simulink model "BatteryHVDetailed_harness_model"  (R2022a)
settings: Solver=daessc  StartTime=0.0  StopTime=500  RelTol=1e-3  AbsTol=1e-3
PreLoadFcn:
  | BatteryHVDetailed_harness_params
  | 
  | load("BatteryHV_CurrentProfile.mat")
undefined symbols (not defined in the file or in its folder): Module, Multi
libraries: fl_lib x2, nesl_utility x2
settings Model: PacingRate=6  Creator=isaacito  LastModifiedBy=isaacito
settings SolverCC: AutoScaleAbsTol=off  AlgebraicLoopSolver=TrustRegion
settings DataIOCC: DSMLogging=off
settings DebuggingCC: UnconnectedInputMsg=warning  UnconnectedOutputMsg=warning  UnconnectedLineMsg=warning  SFMachineParentedDataDiag=warning
settings RTWCC: DLArmComputeVersion=19.05
settings SimscapeCC: SimscapeLogType=local  SimscapeLogSimulationStatistics=on  SimscapeLogToSDI=on  SimscapeLogLimitData=off

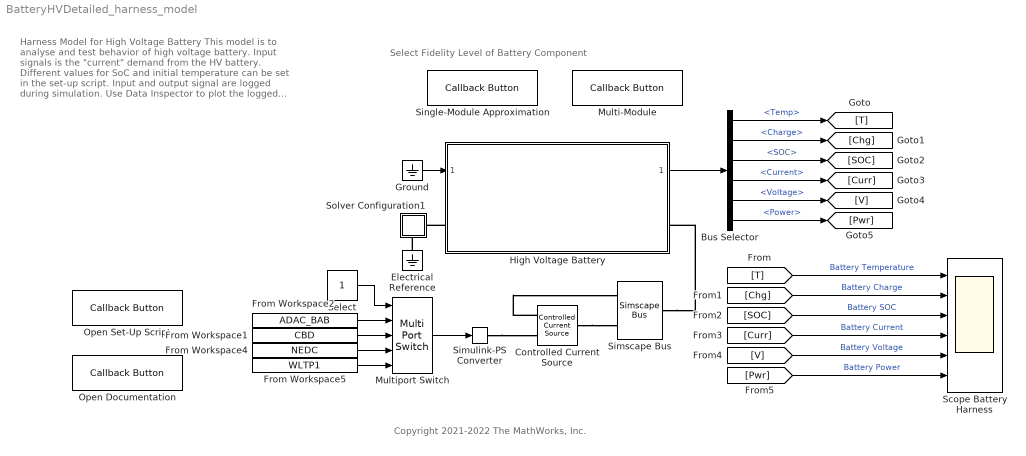
== system BatteryHVDetailed_harness_model ==
  note: Select Fidelity Level of Battery Component
  note: Copyright 2021-2022 The MathWorks, Inc.
  note: Harness Model for
      | High Voltage Battery
      |
      | This model is to analyse and test behavior of high voltage battery.
      |
      | Input signals is the "current" demand from the HV battery. Different values for SoC and initial temperature can be set in the set-up script.
      |
      | Input and output signal are logged during simulation. Use Data Inspector to plot the logged signals.
  " Simscape Bus" : SimscapeBus  HierarchyStrings=plus;minus
  Bus Selector : BusSelector  OutputSignals=Temp,Charge,SOC,Current,Voltage,Power
  Controlled Current Source : fl_lib/Electrical/Electrical Sources/Controlled Current Source
      settings: SourceProductBaseCode=PW,SS,VE
  Electrical Reference : fl_lib/Electrical/Electrical Elements/Electrical Reference
      settings: SourceProductBaseCode=PW,SS,VE
  From Workspace1 : FromWorkspace  VariableName=CBD
  From Workspace2 : FromWorkspace  VariableName=ADAC_BAB
  From Workspace4 : FromWorkspace  VariableName=NEDC
  From Workspace5 : FromWorkspace  VariableName=WLTP1
  Ground : Ground
  High Voltage Battery : Subsystem  ReferencedSubsystem=BatteryHVDetailed_refsub_SingleApprox
  Multi-Module : CallbackButton  ButtonText=Multi-Module
      settings: ClickFcn=|
      | disp("Selecting " + ...
      |   "multi-module component...")
      | 
      | set_param( gcs + "/High Voltage Battery", ...
      |   ReferencedSubsystem = ...
      |   "BatteryHVDetailed_refsub_MultiModule");
      | 
      | BatteryHVDetailed_params_MultiModule
      | 
      | load("BatteryHV_CurrentProfile.mat")
  Multiport Switch : MultiPortSwitch  Inputs=4  SaturateOnIntegerOverflow=off  InputSameDT=off
  Open Documentation : CallbackButton  ButtonText=Open Doc
      settings: ClickFcn=open('batteryModuleDoc_parameterDefinition.html')
  Open Set-Up Script : CallbackButton  ButtonText=Open Script
      settings: ClickFcn="edit(\"BatteryHVDetailed_harness_params\")"
  Scope Battery Harness : Scope  NumInputPorts=6
  Select : Constant
  Simulink-PS Converter : nesl_utility/Simulink-PS Converter  PhysicalDomain=network_engine_domain  SubClassName=ps_input  LeftPortType=input  RightPortType=output  PseudoPeriodic=off  Frequencies=[]  NoiseDistribution=none  NoiseParameters=[]  Unit=A  AffineConversion=off  FilteringAndDerivatives=provide  SimscapeFilterOrder=1  InputFilterTimeConstant=0.001  UdotUserProvided=0
      settings: SourceProductBaseCode=SS,PW,VE
  Single-Module Approximation : CallbackButton  ButtonText=Single-Module Approx.
      settings: ClickFcn=|
      | disp("Selecting " + ...
      |   "single-module approximation component...")
      | 
      | set_param( gcs + "/High Voltage Battery", ...
      |   ReferencedSubsystem = ...
      |   "BatteryHVDetailed_refsub_SingleApprox");
      | 
      | BatteryHVDetailed_params_SingleApprox
      | 
      | load("BatteryHV_CurrentProfile.mat")
  Solver Configuration1 : Subsystem
      settings: PortSchema="{\"entries\":[{\"content\":{\"sides\":[{\"content\":{\"connectorIds\":[]},\"type\":\"ConnectorPlacement.EquallySpacedRectSide\",\"uuid\":\"4a7e26c2-e9e9-4fea-b605-533b1a682be7\"},{\"content\":{\"connectorIds\":[\"RConn1\"],\"side\":\"RIGHT\"},\"type\":\"ConnectorPlacement.EquallySpacedRectSide\",\"uuid\":\"0210e324-555e-4372-b836-fcc8ab23e933\"},{\"content\":{\"connectorIds\":[],\"side\":\"TOP\"},\"type\":\"ConnectorPlacement.EquallySpacedRectSide\",\"uuid\":\"9bbae011-e6fc-4534-a44f-d79a5697c939\"},{\"content\":{\"connectorIds\":[\"RConn2\"],\"side\":\"BOTTOM\"},\"type\":\"ConnectorPlacement.EquallySpacedRectSide\",\"uuid\":\"d5829c0a-26ea-402d-a1c6-900997ddf1a8\"}]},\"type\":\"ConnectorPlacement.EquallySpacedConnector\",\"uuid\":\"f4e17c65-54c6-42fe-a467-9c6b014b697a\"}],\"packageUris\":[\"http://schema.mathworks.com/mf0/Connector/19700101\"],\"version\":\"1.0\"}"
  wires:
  Multiport Switch/1 -> Simulink-PS Converter/1
  From Workspace1/1 -> Multiport Switch/3
  From Workspace5/1 -> Multiport Switch/5
  From Workspace2/1 -> Multiport Switch/2
  Select/1 -> Multiport Switch/1
  From Workspace4/1 -> Multiport Switch/4
  Ground/1 -> High Voltage Battery/1
  High Voltage Battery/1 -> Bus Selector/1
  Bus Selector/1 -> [T]  "<Temp>"
  Bus Selector/2 -> [Chg]  "<Charge>"
  Bus Selector/3 -> [SOC]  "<SOC>"
  Bus Selector/4 -> [Curr]  "<Current>"
  Bus Selector/5 -> [V]  "<Voltage>"
  Bus Selector/6 -> [Pwr]  "<Power>"
  [T] -> Scope Battery Harness/1  "Battery Temperature"
  [Chg] -> Scope Battery Harness/2  "Battery Charge"
  [SOC] -> Scope Battery Harness/3  "Battery SOC"
  [Curr] -> Scope Battery Harness/4  "Battery Current"
  [V] -> Scope Battery Harness/5  "Battery Voltage"
  [Pwr] -> Scope Battery Harness/6  "Battery Power"
  connections:
  Electrical Reference/LConn1 -- Solver Configuration1/RConn2
  High Voltage Battery/LConn1 -- Solver Configuration1/RConn1
  " Simscape Bus"/RConn1 -- High Voltage Battery/RConn1
  Controlled Current Source/RConn2 -- " Simscape Bus"/LConn1
  Simulink-PS Converter/RConn1 -- Controlled Current Source/RConn1
  Controlled Current Source/LConn1 -- " Simscape Bus"/LConn2

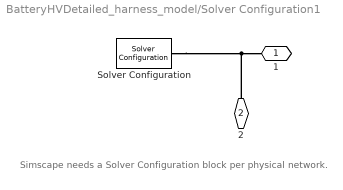
== system BatteryHVDetailed_harness_model/Solver Configuration1 ==
  note: Simscape needs a Solver Configuration block per physical network.
  Solver Configuration : nesl_utility/Solver Configuration  PhysicalDomain=network_engine_domain  SubClassName=solver  LeftPortType=input  RightPortType=generic  Tones=[]  Harmonics=[]  SimulateNoise=off  Profile=off  UseLocalSampling=off  EnableSwitchedLinearOptims=on  FrequencyDomain=off  UseCCode=off  RelTol=0.001  AbsTol=1e-06  MinStep=1e-09  ToWorkspace=off  RevertToSquareIcSolve=off  NumHomotopyIterations=100  PhasorMode=off  PhasorModeNumHarmonics=1  IndexReductionMethod=DerivativeReplacement  DoDC=off  ResidualTolerance=1e-9  UseLocalSolver=off  LocalSolverChoice=NE_BACKWARD_EULER_ADVANCER  LocalSolverSampleTime=0.01  DoFixedCost=off  MaxNonlinIter=3  MaxModeIter=2  ComputeImpulses=off  ImpulseIterations=2  LinearAlgebra=auto  LinearAlgebraNumThread=0  EquationFormulation=NE_TIME_EF  DelaysMemoryBudget=1024  AutomaticFiltering=on  FilteringTimeConstant=0.001  PartitionStorageMethod=AS_NEEDED  PartitionMemoryBudget=1024  PartitionMethod=FAST
      settings: AttributesFormatString=Local solver %<UseLocalSolver>  SourceProductBaseCode=SS,PW,VE
  1 : PMIOPort  Side=Right
  2 : PMIOPort  Port=2  Side=Right
  connections:
  Solver Configuration/RConn1 -- 1/RConn1 -- 2/RConn1
